simulink model "rtwdemo_PCG_Eval_P1"  (Simulink 7.6)
settings: Solver=FixedStepDiscrete  SolverMode=SingleTasking  StartTime=0.0  StopTime=2  FixedStep=.001  MaxStep=10  RelTol=1e-3
PostLoadFcn:
  | if (exist('PCG_Demo_1_data','file'))
  |    load PCG_Demo_1_data;
  | else
  |    % Load Data Objects
  |    RTWDemos.PCG_Eval_Base_Data_Stage_1;
  | end
libraries: rtwdemo_pi_controller x2
CloseFcn:
  | rtwprivate ssgencode ModelCloseRequest rtwdemo_PCG_Eval_P1
settings Model: Creator=The MathWorks Inc.  ExtModeAutoUpdateStatusClock=off
settings SolverCC: InsertRTBMode=Auto
settings DataIOCC: LimitDataPoints=off  SaveFormat=StructureWithTime  SaveOutput=off  SaveTime=off
settings OptimizationCC: InlineParams=on  StateBitsets=on  DataBitsets=on  UseTempVars=on  ZeroExternalMemoryAtStartup=off  ZeroInternalMemoryAtStartup=off  NoFixptDivByZeroProtection=on  EfficientFloat2IntCast=on  OptimizeModelRefInitCode=on  LifeSpan=1
settings DebuggingCC: CheckExecutionContextPreStartOutputMsg=on  CheckExecutionContextRuntimeOutputMsg=on  IntegerOverflowMsg=none  InvalidFcnCallConnMsg=warning  BusObjectLabelMismatch=error  RootOutportRequireBusObject=error  ModelReferenceIOMsg=error  ModelReferenceIOMismatchMessage=error  ModelReferenceCSMismatchMessage=error  ModelReferenceDataLoggingMessage=error
settings HardwareCC: ProdHWDeviceType=32-bit Embedded Processor
settings ModelReferenceCC: ModelReferenceNumInstancesAllowed=Single
settings SFSimCC: SimCustomHeaderCode="#include \"ThrottleBus.h\""  SimUserIncludeDirs="\"$matlabroot$\\toolbox\\rtw\\rtwdemos\\EmbeddedCoderOverview\\\""  SimParseCustomCode=off
settings RTWCC: SystemTargetFile=ert.tlc  GenCodeOnly=on  TemplateMakefile=ert_default_tmf  Description=Real-Time Workshop Embedded Coder (no auto configuration)  GenerateReport=on  ProcessScript=ert_make_rtw_hook  CustomHeaderCode="#include \"ThrottleBus.h\""  IncludeHyperlinkInReport=on
settings CodeAppCC: ForceParamTrailComments=on
settings ERTTargetCC: TargetFcnLib=ansi_tfl_tmw_new.mat  UtilityFuncGeneration=Shared location  MultiwordLength=2048  GenerateSampleERTMain=on  IncludeMdlTerminateFcn=off  SupportAbsoluteTime=off  SupportNonFinite=off  SupportComplex=off  InlinedParameterPlacement=NonHierarchical  ERTCustomFileTemplate=example_file_process.tlc  GlobalDataDefinition=InSeparateSourceFile  DataDefinitionFile=global_data.c  GlobalDataReference=InSeparateHeaderFile  DataReferenceFile=global_data.h  ConvertIfToSwitch=off  EnableUserReplacementTypes=on  MemSecPackage=Simulink  MemSecDataConstants=MemConst

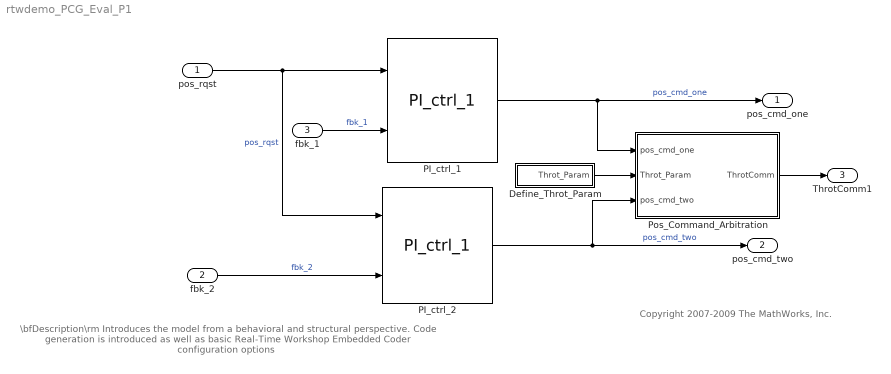
== system rtwdemo_PCG_Eval_P1 ==
  note: Copyright 2007-2009 The MathWorks, Inc.
  note: \bfDescription\rm
      | Introduces the model from a behavioral and structural perspective.  Code generation
      | is introduced as well as basic Real-Time Workshop Embedded Coder configuration
      | options
  pos_rqst : Inport
  fbk_2 : Inport  Port=2
  fbk_1 : Inport  Port=3
  Define_Throt_Param : Subsystem
  PI_ctrl_1 : rtwdemo_pi_controller/PI_ctrl_1  SystemSampleTime=-1
  PI_ctrl_2 : rtwdemo_pi_controller/PI_ctrl_1  SystemSampleTime=-1
  Pos_Command_Arbitration : Stateflow chart  TreatAsAtomicUnit=on
      settings: RTWFcnNameOpts=Use subsystem name  RTWFileNameOpts=Use subsystem name
  pos_cmd_one : Outport
  pos_cmd_two : Outport  Port=2
  ThrotComm1 : Outport  Port=3  OutDataTypeStr=Bus: ThrottleCommands
  wires:
  fbk_1/1 -> PI_ctrl_1/2  "fbk_1"
  pos_rqst/1 -> PI_ctrl_1/1, PI_ctrl_2/1  "pos_rqst"
  fbk_2/1 -> PI_ctrl_2/2  "fbk_2"
  PI_ctrl_1/1 -> pos_cmd_one/1, Pos_Command_Arbitration/1(pos_cmd_one)  "pos_cmd_one"
  PI_ctrl_2/1 -> pos_cmd_two/1, Pos_Command_Arbitration/3(pos_cmd_two)  "pos_cmd_two"
  Pos_Command_Arbitration/1(ThrotComm) -> ThrotComm1/1
  Define_Throt_Param/1(Throt_Param) -> Pos_Command_Arbitration/2(Throt_Param)

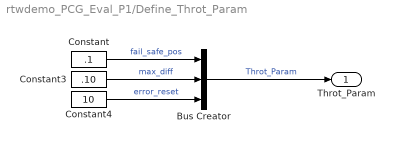
== system rtwdemo_PCG_Eval_P1/Define_Throt_Param ==
  Bus Creator : BusCreator  Inputs=3  OutDataTypeStr=Bus: ThrottleParams  NonVirtualBus=on
  Constant : Constant  Value=.1  OutDataTypeStr=double
  Constant3 : Constant  Value=.10  OutDataTypeStr=double
  Constant4 : Constant  Value=10  OutDataTypeStr=double
  Throt_Param : Outport
  wires:
  Constant/1 -> Bus Creator/1  "fail_safe_pos"
  Constant3/1 -> Bus Creator/2  "max_diff"
  Constant4/1 -> Bus Creator/3  "error_reset"
  Bus Creator/1 -> Throt_Param/1  "Throt_Param"

== stateflow chart Pos_Command_Arbitration ==
  note: The Stateflow Diagram implements an if / elseif / else
  note: End of the if structure
  note: The throttle command signals are not in agreement. Enter into fail safe mode
  note: Not in an error mode:
      | The control signal is selected from the input signal that
      | most closely  matches the last pass value of the signal
  note: The signals have not been in agreement for a
      | long enough time to exit the failure mode: increment the failure counter
  note: Enough time has passed to exit the failure mode:
      | reset the mode and the counter
  (default) -> (junction 18) : {
      |  ThrotComm.pos_cmd_raw[0] = pos_cmd_one;...
      |  ThrotComm.pos_cmd_raw[1] = pos_cmd_two;
      | }
  (junction 18) -> (junction 10) [order 1] : [abs(pos_cmd_one - pos_cmd_two) > Throt_Param.max_diff]
  (junction 9) -> (junction 11) [order 2]
  (junction 17) -> (junction 12) : {
      | ThrotComm.pos_failure_mode = 0;
      | ThrotComm.err_cnt = 0;
      | }
  (junction 19) -> (junction 16) [order 1] : [ThrotComm.pos_failure_mode > 0]
  (junction 14) -> (junction 15)
  (junction 19) -> (junction 22) [order 2]
  (junction 10) -> (junction 21) : {
      |  ThrotComm.pos_failure_mode = 1;...
      |  ThrotComm.err_cnt = 0;
      |  ThrotComm.pos_cmd_act = Throt_Param.fail_safe_pos;
      | }
  (junction 9) -> (junction 17) [order 1] : [ThrotComm.err_cnt >= Throt_Param.error_reset]
  (junction 18) -> (junction 9) [order 2]
  (junction 16) -> (junction 20) : {
      |  ThrotComm.err_cnt++;
      | }
  (junction 22) -> (junction 14) [order 2] : {
      | ThrotComm.pos_cmd_act = pos_cmd_two;
      | }
  (junction 12) -> (junction 11)
  (junction 22) -> (junction 23) [order 1] : [abs(pos_cmd_one - ThrotComm.pos_cmd_act) < ...
      | abs(pos_cmd_two - ThrotComm.pos_cmd_act)]
  (junction 23) -> (junction 13) : {
      | ThrotComm.pos_cmd_act = pos_cmd_one;
      | }
  (junction 11) -> (junction 19)
  (junction 21) -> (junction 20)
  (junction 20) -> (junction 13)
  (junction 13) -> (junction 14)
  data: pos_cmd_one input double; Throt_Param input Bus: ThrottleParams size=1; pos_cmd_two input double; ThrotComm output Bus: ThrottleCommands size=1; fail_safe_pos local double =.1
